simulink model "q1_sim"  (R2019b)
settings: Solver=VariableStepAuto  StartTime=0.0  StopTime=50  RelTol=1e-3
settings Model: Creator=Mertcan  LastModifiedBy=Mertcan

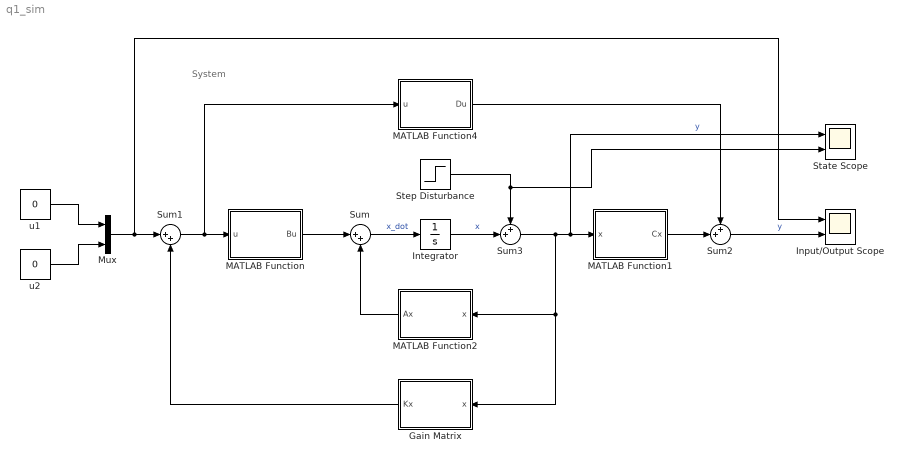
== system q1_sim ==
  note: System
  Gain Matrix : MATLAB Function  TreatAsAtomicUnit=on
  Input/Output Scope : Scope  NumInputPorts=2
  Integrator : Integrator
  MATLAB Function : MATLAB Function  TreatAsAtomicUnit=on
  MATLAB Function1 : MATLAB Function  TreatAsAtomicUnit=on
  MATLAB Function2 : MATLAB Function  TreatAsAtomicUnit=on
  MATLAB Function4 : MATLAB Function  TreatAsAtomicUnit=on
  Mux : Mux  Inputs=2
  State Scope : Scope  NumInputPorts=2
  Step Disturbance : Step  After=0.1  SampleTime=0
  Sum : Sum  Inputs=|++
  Sum1 : Sum  Inputs=|++
  Sum2 : Sum  Inputs=++|
  Sum3 : Sum  Inputs=++|
  u1 : Constant  Value=0
  u2 : Constant  Value=0
  wires:
  MATLAB Function/1(Bu) -> Sum/1
  Sum/1 -> Integrator/1  "x_dot"
  MATLAB Function2/1(Ax) -> Sum/2
  Sum1/1 -> MATLAB Function4/1(u), MATLAB Function/1(u)
  Gain Matrix/1(Kx) -> Sum1/2
  MATLAB Function1/1(Cx) -> Sum2/2
  MATLAB Function4/1(Du) -> Sum2/1
  Sum2/1 -> Input/Output Scope/2  "y"
  Mux/1 -> Input/Output Scope/1, Sum1/1
  u1/1 -> Mux/1
  u2/1 -> Mux/2
  Integrator/1 -> Sum3/2  "x"
  Sum3/1 -> Gain Matrix/1(x), MATLAB Function2/1(x), State Scope/1, MATLAB Function1/1(x)  "y"
  Step Disturbance/1 -> State Scope/2, Sum3/1

== matlab function q1_sim/MATLAB Function1 ==
  data: x input; Cx output
function Cx = Cmat(x)

C = [0 1 0 0
    0 0 0 1];

Cx = C*x;

== matlab function q1_sim/MATLAB Function ==
  data: u input; Bu output
function Bu = Bmat(u)

B = [0.094 -2.169
    0 0.038
    0.611 1.190
    0 0];

Bu = B*u;

== matlab function q1_sim/MATLAB Function2 ==
  data: x input; Ax output
function Ax = Amat(x)

A = [-0.275 2.682 0.0067 0
    -0.994 -0.125 -0.003 0.074
    0.365 -6.695 -1.004 0
    -0.002 0 1 0];

Ax = A*x;

== matlab function q1_sim/Gain Matrix ==
  data: x input; Kx output
function Kx = Kmat(x)

K = [-0.262316, 8.31301, 1.58143, 0.0617323
    -3.34649, -0.0898956, -7.16616, -0.250465];

Kx = K*x;

== matlab function q1_sim/MATLAB Function4 ==
  data: u input; Du output
function Du = Dmat(u)

D = [0 0
    0 0];

Du = D*u;
